simulink model "Problem3"  (R2020b)
settings: Solver=VariableStepAuto  StartTime=0.0  StopTime=10.0  RelTol=1e-3
settings Model: Creator=Dell  LastModifiedBy=Dell

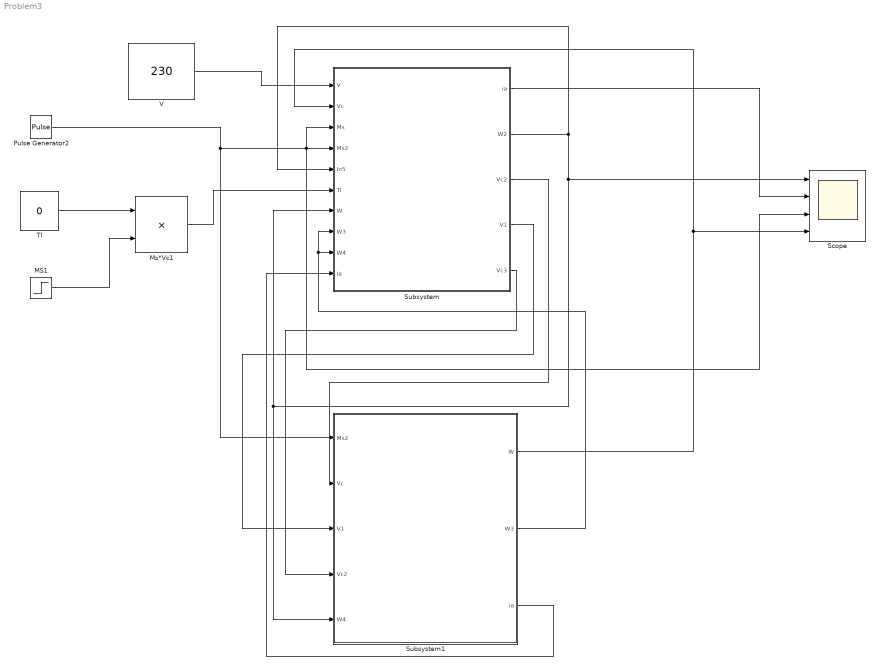
== system Problem3 ==
  MS1 : Step  Time=20  SampleTime=0
  Ms*Vc1 : Product
  Pulse Generator2 : DiscretePulseGenerator  PulseType=Time based  Period=90  PulseWidth=95
  Scope : Scope  NumInputPorts=4
  Subsystem : Subsystem
  Subsystem1 : Subsystem
  Tl : Constant  Value=0
  V : Constant  Value=230
  wires:
  Pulse Generator2/1 -> Subsystem1/1(Ms2), Scope/3, Subsystem/3(Ms), Subsystem/4(Ms2)
  Tl/1 -> Ms*Vc1/1
  Ms*Vc1/1 -> Subsystem/6(Tl)
  Subsystem/3(Vc2) -> Subsystem1/2(Vc)
  Subsystem/1(ia) -> Scope/2
  MS1/1 -> Ms*Vc1/2
  V/1 -> Subsystem/1(V)
  Subsystem/4(V1) -> Subsystem1/3(V1)
  Subsystem1/2(W3) -> Subsystem/8(W3), Subsystem/9(W4)
  Subsystem/5(Vc3) -> Subsystem1/4(Vc2)
  Subsystem1/1(W) -> Scope/4, Subsystem/2(Vc)
  Subsystem1/3(ia) -> Subsystem/10(Ia)
  Subsystem/2(W2) -> Subsystem1/5(W4), Subsystem/7(W), Scope/1, Subsystem/5(In5)

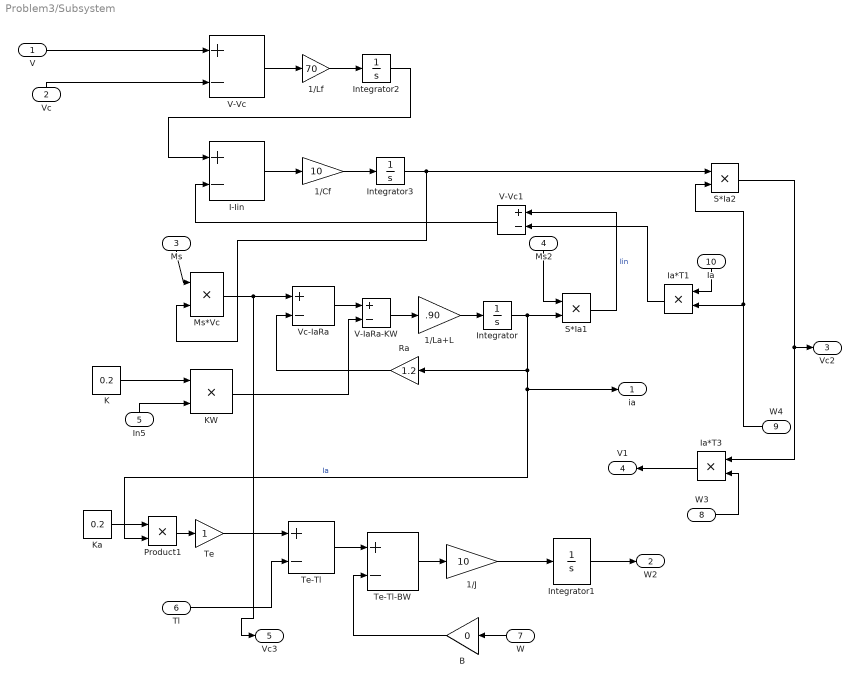
== system Problem3/Subsystem ==
  V : Inport
  Vc : Inport  Port=2
  Ms : Inport  Port=3
  Ms2 : Inport  Port=4
  In5 : Inport  Port=5
  Tl : Inport  Port=6
  W : Inport  Port=7
  W3 : Inport  Port=8
  W4 : Inport  Port=9
  Ia : Inport  Port=10
  1/Cf : Gain  Gain=10
  1/J : Gain  Gain=10
  1/La+L : Gain  Gain=.90
  1/Lf : Gain  Gain=70
  B : Gain  Gain=0
  I-Iin : Sum  Inputs=+-
  Ia*T1 : Product
  Ia*T3 : Product
  Integrator{,1..3} (4 alike) : Integrator
  K : Constant  Value=0.2
  KW : Product
  Ka : Constant  Value=0.2
  Ms*Vc : Product
  Product1 : Product
  Ra : Gain  Gain=1.2
  S*Ia1 : Product
  S*Ia2 : Product
  Te : Gain
  Te-Tl : Sum  Inputs=+-
  Te-Tl-BW : Sum  Inputs=+-
  V-IaRa-KW : Sum  Inputs=+-
  V-Vc : Sum  Inputs=+-
  V-Vc1 : Sum  Inputs=+-
  Vc-IaRa : Sum  Inputs=+-
  ia : Outport
  W2 : Outport  Port=2
  Vc2 : Outport  Port=3
  V1 : Outport  Port=4
  Vc3 : Outport  Port=5
  wires:
  Product1/1 -> Te/1
  K/1 -> KW/1
  Te-Tl-BW/1 -> 1/J/1
  Ra/1 -> Vc-IaRa/2
  V-Vc/1 -> 1/Lf/1
  B/1 -> Te-Tl-BW/2
  Vc-IaRa/1 -> V-IaRa-KW/1
  Integrator/1 -> Product1/2, ia/1, Ra/1, S*Ia1/2  "Ia"
  Te/1 -> Te-Tl/1
  1/J/1 -> Integrator1/1
  KW/1 -> V-IaRa-KW/2
  1/Cf/1 -> Integrator3/1
  1/La+L/1 -> Integrator/1
  Integrator2/1 -> I-Iin/1
  1/Lf/1 -> Integrator2/1
  V-IaRa-KW/1 -> 1/La+L/1
  Ka/1 -> Product1/1
  Te-Tl/1 -> Te-Tl-BW/1
  Ia*T3/1 -> V1/1
  Tl/1 -> Te-Tl/2
  Ms*Vc/1 -> Vc3/1, Vc-IaRa/1
  Integrator3/1 -> S*Ia2/1, Ms*Vc/2
  S*Ia1/1 -> V-Vc1/1  "Iin"
  V/1 -> V-Vc/1
  Ia*T1/1 -> V-Vc1/2
  I-Iin/1 -> 1/Cf/1
  V-Vc1/1 -> I-Iin/2
  S*Ia2/1 -> Vc2/1, Ia*T3/1
  Integrator1/1 -> W2/1
  W/1 -> B/1
  Vc/1 -> V-Vc/2
  W3/1 -> Ia*T3/2
  Ms2/1 -> S*Ia1/1
  Ia/1 -> Ia*T1/1
  In5/1 -> KW/2
  W4/1 -> S*Ia2/2, Ia*T1/2
  Ms/1 -> Ms*Vc/1

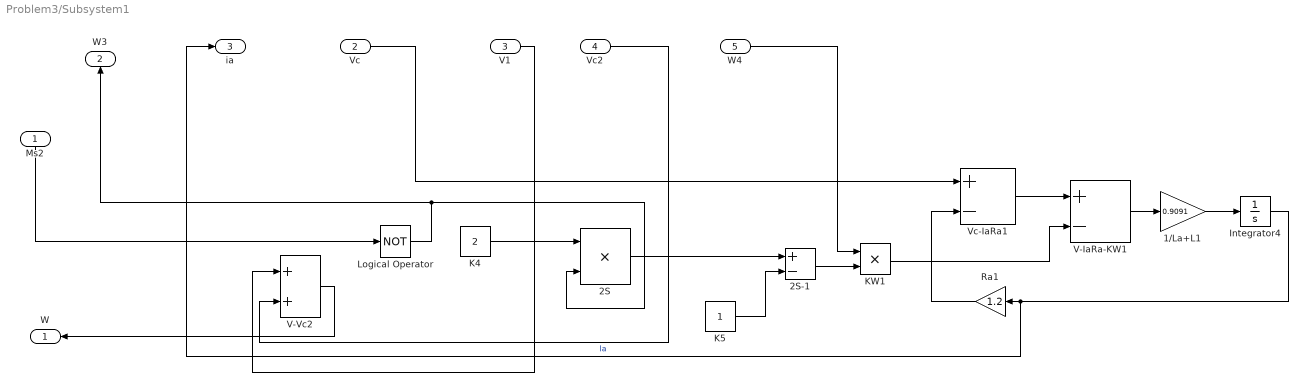
== system Problem3/Subsystem1 ==
  Ms2 : Inport
  Vc : Inport  Port=2
  V1 : Inport  Port=3
  Vc2 : Inport  Port=4
  W4 : Inport  Port=5
  1/La+L1 : Gain  Gain=0.9091
  2S : Product
  2S-1 : Sum  Inputs=+-
  Integrator4 : Integrator
  K4 : Constant  Value=2
  K5 : Constant
  KW1 : Product
  Logical Operator : Logic  Operator=NOT  AllPortsSameDT=off  OutDataTypeStr=boolean
  Ra1 : Gain  Gain=1.2
  V-IaRa-KW1 : Sum  Inputs=+-
  V-Vc2 : Sum
  Vc-IaRa1 : Sum  Inputs=+-
  W : Outport
  W3 : Outport  Port=2
  ia : Outport  Port=3
  wires:
  W4/1 -> KW1/1
  Ms2/1 -> Logical Operator/1
  Vc2/1 -> V-Vc2/2
  Vc/1 -> Vc-IaRa1/1
  V1/1 -> V-Vc2/1
  V-Vc2/1 -> W/1
  V-IaRa-KW1/1 -> 1/La+L1/1
  Integrator4/1 -> ia/1, Ra1/1  "Ia"
  KW1/1 -> V-IaRa-KW1/2
  Logical Operator/1 -> W3/1, 2S/2
  K5/1 -> 2S-1/2
  2S/1 -> 2S-1/1
  K4/1 -> 2S/1
  Vc-IaRa1/1 -> V-IaRa-KW1/1
  Ra1/1 -> Vc-IaRa1/2
  1/La+L1/1 -> Integrator4/1
  2S-1/1 -> KW1/2
